simulink model "buck_hvoltage"  (Simulink 8.3)
settings: Solver=ode45  StartTime=0.0  StopTime=Tmax  RelTol=1e-3
values from neighbouring files (symbols this model uses):
  a00c = sys(1).Ac(1,1)    [parameters.m]
  a00o = sys(1).Ao(1,1)    [parameters.m]
  a01c = sys(1).Ac(1,2)    [parameters.m]
  a01o = sys(1).Ao(1,2)    [parameters.m]
  a10c = sys(1).Ac(2,1)    [parameters.m]
  a10o = sys(1).Ao(2,1)    [parameters.m]
  a11c = sys(1).Ac(2,2)    [parameters.m]
  a11o = sys(1).Ao(2,2)    [parameters.m]
  b0c = sys(1).Bc(1)    [parameters.m]
  b0o = sys(1).Bo(1)    [parameters.m]
  b1c = sys(1).Bc(2)    [parameters.m]
  b1o = sys(1).Bo(2)    [parameters.m]
  D = cr*Vref/(cr*Vref + Vs)    (= 0.489795918367)    [parameters.m]
  i0 = 4.5    [parameters.m]
  T = 4e-6    (= 4e-06)    [parameters.m]
  v0 = 48    [parameters.m]
  Vref = 15    [parameters.m]    (also in parameters_dcmicrogrid.m = [48 48]; parameters_dcmicrogrid_hynger.m = [48 48])
  Vtol = Vref / 200    (= 0.075)    [parameters.m]
settings Model: Creator=Luan Nguyen  LastModifiedBy=tjohnson
settings OptimizationCC: ExpressionDepthLimit=2147483647
settings DebuggingCC: MaxConsecutiveZCsMsg=none  MultiTaskDSMMsg=warning  MultiTaskCondExecSysMsg=none  FrameProcessingCompatibilityMsg=error
settings GRTTargetCC: CombineOutputUpdateFcns=on  GRTInterface=off

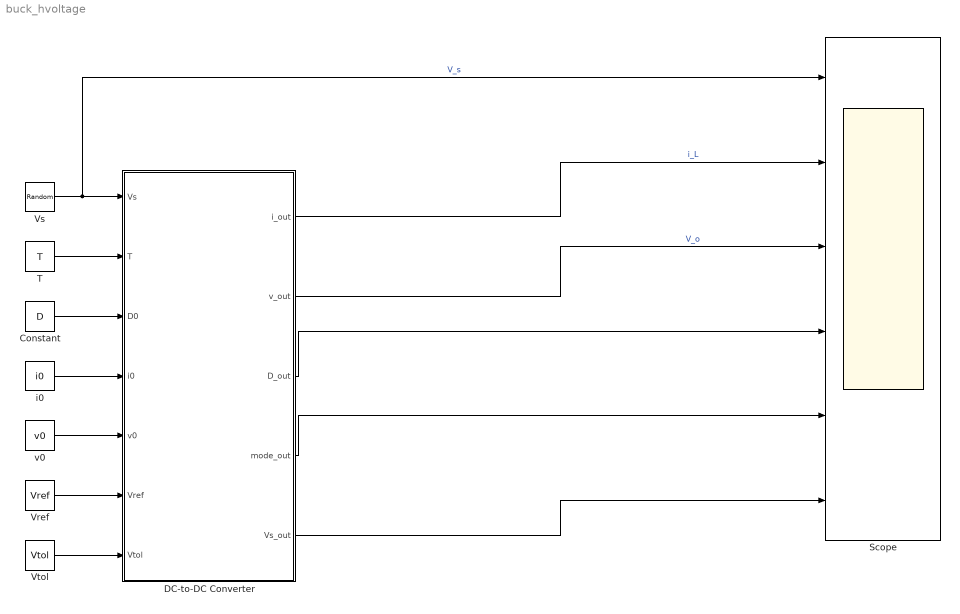
== system buck_hvoltage ==
  Constant : Constant  Value=D
  DC-to-DC Converter : Stateflow chart  TreatAsAtomicUnit=on
      settings: PermitHierarchicalResolution=ParametersOnly
  Scope : Scope  NumInputPorts=6
      settings: TimeRange=0.03  YMin=85~-0.5~47.65~0.57684~1~85  YMax=112.5~9.5~48.45~0.63756~3~112.5  SaveName=dc2dc_ScopeData
  T : Constant  Value=T
  Vref : Constant  Value=Vref
  Vs : RandomNumber  Mean=100  Variance=100  SampleTime=T*100
  Vtol : Constant  Value=Vtol
  i0 : Constant  Value=i0
  v0 : Constant  Value=v0
  wires:
  DC-to-DC Converter/1(i_out) -> Scope/2  "i_L"
  DC-to-DC Converter/2(v_out) -> Scope/3  "V_o"
  T/1 -> DC-to-DC Converter/2(T)
  Vs/1 -> Scope/1, DC-to-DC Converter/1(Vs)  "V_s"
  i0/1 -> DC-to-DC Converter/4(i0)
  v0/1 -> DC-to-DC Converter/5(v0)
  Constant/1 -> DC-to-DC Converter/3(D0)
  Vref/1 -> DC-to-DC Converter/6(Vref)
  DC-to-DC Converter/3(D_out) -> Scope/4
  DC-to-DC Converter/4(mode_out) -> Scope/5
  Vtol/1 -> DC-to-DC Converter/7(Vtol)
  DC-to-DC Converter/5(Vs_out) -> Scope/6

== stateflow chart DC-to-DC Converter ==
  settings: updateMethod=CONTINUOUS
  state Discontinuous
    du:
    i_dot = a00d*i+a01d*v+b0d*Vs;
    v_dot = a10d*i+a11d*v+b1d*Vs;
    t_dot = 1;
    i_out =i;
    v_out = v;
    D_out=D;
    mode_out=3;
    Vs_out=Vs;
  state Charging
    du:
    i_dot = a00c*i+a01c*v+b0c*Vs;
    v_dot = a10c*i+a11c*v+b1c*Vs;
    t_dot = 1;
    i_out = i;
    v_out = v;
    D_out=D;
    mode_out=2;
    Vs_out=Vs;
  state Discharging
    du:
    i_dot = a00o*i+a01o*v+b0o*Vs;
    v_dot = a10o*i+a11o*v+b1o*Vs;
    t_dot = 1;
    i_out = i;
    v_out = v;
    D_out=D;
    mode_out=1;
    Vs_out=Vs;
  Discharging -> Discontinuous [order 1] : [i<=0]
  Discontinuous -> Charging : [t>=(1-D)*T]
      | {t=0;}
  Charging -> Discharging : [v>=(Vref+Vtol)&&t>=D*T]
      | {t= 0;}
  Discharging -> Charging [order 2] : [v<=(Vref-Vtol)&&t>=(1-D)*T]
      | {t= 0;}
  (default) -> Charging : {i = i0;
      | v = v0;
      | D=D0;}
  data: t local double; i_out output double; v_out output double; i local double; a00o local double; Vs input double =120; T input double; D0 input double; a01o local double; a10o local double; a11o local double; a00c local double; a01c local double; a10c local double; a11c local double; b0o local double; b1o local double; b0c local double; b1c local double; v local double; i0 input double; v0 input double; a01d local double; a10d local double; a11d local double; a00d local double; b0d local double; b1d local double; Vref input double =120; D local double; v1 local double; D_out output double; mode_out output double; Vtol input double =120; Vs_out output double
  data t settings: updateMethod=SF_CONTINUOUS_TIME_DATA
  data i settings: updateMethod=SF_CONTINUOUS_TIME_DATA
  data v settings: updateMethod=SF_CONTINUOUS_TIME_DATA
  data D settings: updateMethod=SF_CONTINUOUS_TIME_DATA
  data v1 settings: updateMethod=SF_CONTINUOUS_TIME_DATA
  data Vtol settings: description=Voltage tolerance (e.g., Vref / 100 is +/- 1% voltage ripple)
